simulink model "second_order_algorithm"  (R2020b)
settings: Solver=VariableStepAuto  StartTime=0.0  StopTime=4  RelTol=1e-3
undefined symbols (not defined in the file or in its folder): DiscIntNeverNeededParam
settings Model: Creator=martin  LastModifiedBy=martin

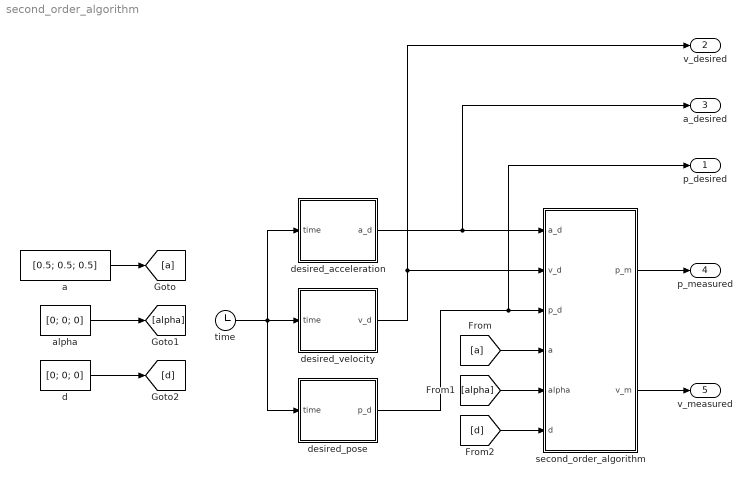
== system second_order_algorithm ==
  a : Constant  Value=[0.5; 0.5; 0.5]
  alpha : Constant  Value=[0; 0; 0]
  d : Constant  Value=[0; 0; 0]
  desired_acceleration : Subsystem
  desired_pose : Subsystem
  desired_velocity : Subsystem
  second_order_algorithm : Subsystem
  time : Clock
  p_desired : Outport
  v_desired : Outport  Port=2
  a_desired : Outport  Port=3
  p_measured : Outport  Port=4
  v_measured : Outport  Port=5
  wires:
  time/1 -> desired_pose/1(time), desired_velocity/1(time), desired_acceleration/1(time)
  a/1 -> [a]
  alpha/1 -> [alpha]
  d/1 -> [d]
  desired_velocity/1(v_d) -> second_order_algorithm/2(v_d), v_desired/1
  desired_pose/1(p_d) -> second_order_algorithm/3(p_d), p_desired/1
  [a] -> second_order_algorithm/4(a)
  [alpha] -> second_order_algorithm/5(alpha)
  [d] -> second_order_algorithm/6(d)
  second_order_algorithm/1(p_m) -> p_measured/1
  second_order_algorithm/2(v_m) -> v_measured/1
  desired_acceleration/1(a_d) -> second_order_algorithm/1(a_d), a_desired/1

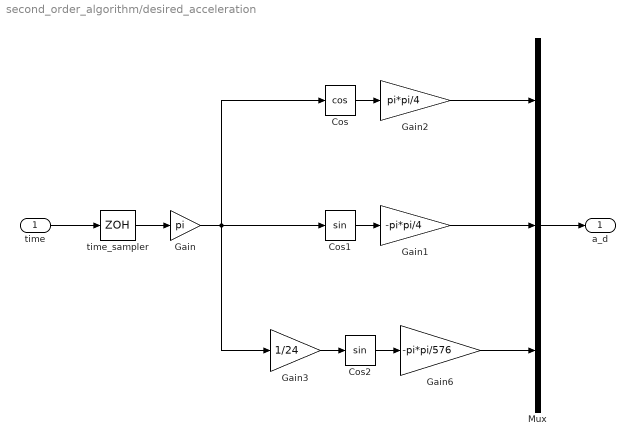
== system second_order_algorithm/desired_acceleration ==
  time : Inport
  Cos : Trigonometry  Operator=cos
  Cos1 : Trigonometry
  Cos2 : Trigonometry
  Gain : Gain  Gain=pi
  Gain1 : Gain  Gain=-pi*pi/4
  Gain2 : Gain  Gain=pi*pi/4
  Gain3 : Gain  Gain=1/24
  Gain6 : Gain  Gain=-pi*pi/576
  Mux : Mux  Inputs=3
  time_sampler : ZeroOrderHold  SampleTime=1e-3
  a_d : Outport
  wires:
  Mux/1 -> a_d/1
  Gain2/1 -> Mux/1
  Gain1/1 -> Mux/2
  time_sampler/1 -> Gain/1
  time/1 -> time_sampler/1
  Gain/1 -> Cos/1, Cos1/1, Gain3/1
  Cos/1 -> Gain2/1
  Cos1/1 -> Gain1/1
  Gain3/1 -> Cos2/1
  Cos2/1 -> Gain6/1
  Gain6/1 -> Mux/3

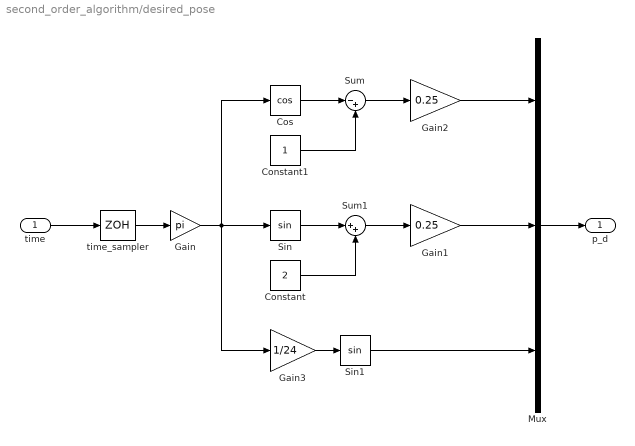
== system second_order_algorithm/desired_pose ==
  time : Inport
  Constant : Constant  Value=2
  Constant1 : Constant
  Cos : Trigonometry  Operator=cos
  Gain : Gain  Gain=pi
  Gain1 : Gain  Gain=0.25
  Gain2 : Gain  Gain=0.25
  Gain3 : Gain  Gain=1/24
  Mux : Mux  Inputs=3
  Sin : Trigonometry
  Sin1 : Trigonometry
  Sum : Sum  Inputs=|-+
  Sum1 : Sum  Inputs=|++
  time_sampler : ZeroOrderHold  SampleTime=1e-3
  p_d : Outport
  wires:
  Mux/1 -> p_d/1
  Cos/1 -> Sum/1
  Sum/1 -> Gain2/1
  Constant1/1 -> Sum/2
  Gain/1 -> Gain3/1, Sin/1, Cos/1
  Sin1/1 -> Mux/3
  Gain2/1 -> Mux/1
  Gain3/1 -> Sin1/1
  Gain1/1 -> Mux/2
  Sin/1 -> Sum1/1
  Constant/1 -> Sum1/2
  Sum1/1 -> Gain1/1
  time_sampler/1 -> Gain/1
  time/1 -> time_sampler/1

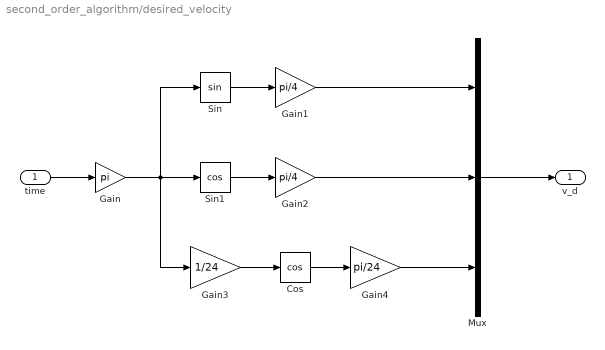
== system second_order_algorithm/desired_velocity ==
  time : Inport
  Cos : Trigonometry  Operator=cos
  Gain : Gain  Gain=pi
  Gain1 : Gain  Gain=pi/4
  Gain2 : Gain  Gain=pi/4
  Gain3 : Gain  Gain=1/24
  Gain4 : Gain  Gain=pi/24
  Mux : Mux  Inputs=3
  Sin : Trigonometry
  Sin1 : Trigonometry  Operator=cos
  v_d : Outport
  wires:
  time/1 -> Gain/1
  Gain/1 -> Gain3/1, Sin1/1, Sin/1
  Sin/1 -> Gain1/1
  Sin1/1 -> Gain2/1
  Gain3/1 -> Cos/1
  Cos/1 -> Gain4/1
  Gain1/1 -> Mux/1
  Gain2/1 -> Mux/2
  Mux/1 -> v_d/1
  Gain4/1 -> Mux/3

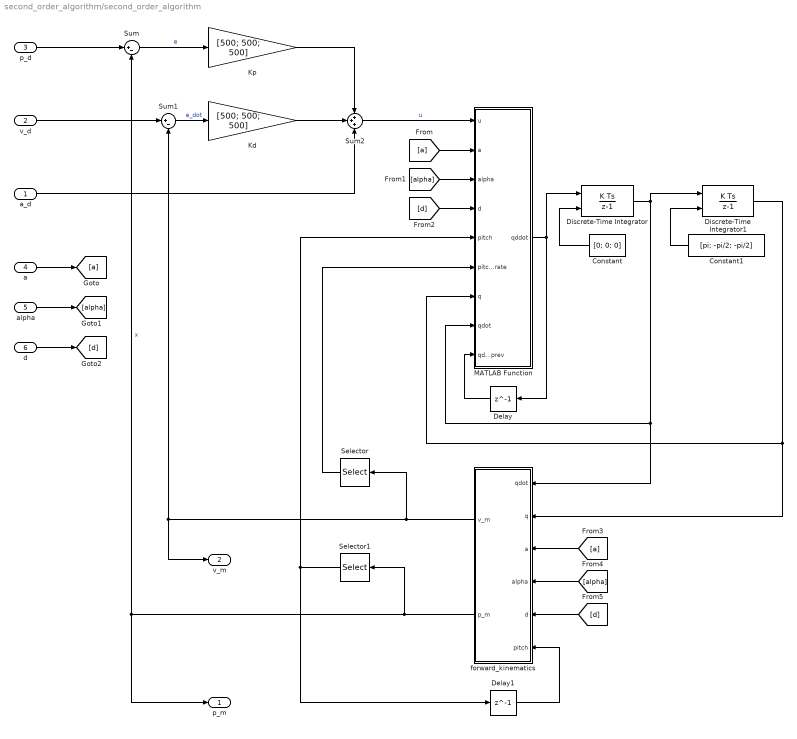
== system second_order_algorithm/second_order_algorithm ==
  a_d : Inport
  v_d : Inport  Port=2
  p_d : Inport  Port=3
  a : Inport  Port=4
  alpha : Inport  Port=5
  d : Inport  Port=6
  Constant : Constant  Value=[0; 0; 0]
  Constant1 : Constant  Value=[pi; -pi/2; -pi/2]
  Delay : Delay  DelayLength=1
  Delay1 : Delay  DelayLength=1
  Discrete-Time Integrator : DiscreteIntegrator  InitialConditionSource=external  SampleTime=1e-3  ICPrevOutput=DiscIntNeverNeededParam  ICPrevScaledInput=DiscIntNeverNeededParam
  Discrete-Time Integrator1 : DiscreteIntegrator  InitialConditionSource=external  SampleTime=1e-3  ICPrevOutput=DiscIntNeverNeededParam  ICPrevScaledInput=DiscIntNeverNeededParam
  Kd : Gain  Gain=[500; 500; 500]
  Kp : Gain  Gain=[500; 500; 500]
  MATLAB Function : MATLAB Function  TreatAsAtomicUnit=on
  Selector : Selector  InputPortWidth=3  IndexOptions=Index vector (dialog)  Indices=[3]  OutputSizes=1
  Selector1 : Selector  InputPortWidth=3  IndexOptions=Index vector (dialog)  Indices=[3]  OutputSizes=1
  Sum : Sum  Inputs=|+-
  Sum1 : Sum  Inputs=|+-
  Sum2 : Sum  Inputs=+++
  forward_kinematics : MATLAB Function  TreatAsAtomicUnit=on
  p_m : Outport
  v_m : Outport  Port=2
  wires:
  [d] -> forward_kinematics/5(d)
  [a] -> forward_kinematics/3(a)
  [alpha] -> forward_kinematics/4(alpha)
  Sum/1 -> Kp/1  "e"
  p_d/1 -> Sum/1
  v_d/1 -> Sum1/1
  Sum1/1 -> Kd/1  "e_dot"
  Kp/1 -> Sum2/1
  a_d/1 -> Sum2/3
  Kd/1 -> Sum2/2
  Sum2/1 -> MATLAB Function/1(u)  "u"
  MATLAB Function/1(qddot) -> Delay/1, Discrete-Time Integrator/1
  Constant/1 -> Discrete-Time Integrator/2
  Discrete-Time Integrator/1 -> forward_kinematics/1(qdot), MATLAB Function/8(qdot), Discrete-Time Integrator1/1
  Constant1/1 -> Discrete-Time Integrator1/2
  [alpha] -> MATLAB Function/3(alpha)
  [a] -> MATLAB Function/2(a)
  [d] -> MATLAB Function/4(d)
  Delay/1 -> MATLAB Function/9(qddot_prev)
  Discrete-Time Integrator1/1 -> forward_kinematics/2(q), MATLAB Function/7(q)
  forward_kinematics/1(v_m) -> Selector/1, v_m/1, Sum1/2
  forward_kinematics/2(p_m) -> Selector1/1, p_m/1, Sum/2  "x"
  Selector/1 -> MATLAB Function/6(pitch_rate)
  Selector1/1 -> Delay1/1, MATLAB Function/5(pitch)
  Delay1/1 -> forward_kinematics/6(pitch)
  alpha/1 -> [alpha]
  a/1 -> [a]
  d/1 -> [d]

== matlab function second_order_algorithm/forward_kinematics ==
  data: v_m output; qdot input; q input; a input; alpha input; d input; p_m output; pitch input
function [v_m, p_m] = fcn(qdot, q, a, alpha, d, pitch)
joint_type = ['r'; 'r'; 'r'];

s = forward_kinematics(joint_type, q, a, alpha, d);

J = s.analytical_jacobian(0, pitch);
J_min = [J(1:2,:); J(6,:)];
v_m = J_min*qdot;

x = s.end_effector_pose();
p_m = [x(1:2,:); x(6,:)];

== matlab function second_order_algorithm/MATLAB Function ==
  data: u input size=[3,1]; a input; alpha input; d input; pitch input; pitch_rate input; qddot output size=[3,1]; q input size=[3,1]; qdot input size=[3,1]; qddot_prev input size=[3,1]
function qddot = fcn(u, a, alpha, d, pitch, pitch_rate, q, qdot, qddot_prev)

joint_type = ['r'; 'r'; 'r'];

s = forward_kinematics(joint_type, q, a, alpha, d);

J = s.analytical_jacobian(0, pitch);

J_min = [J(1:2,:); J(6,:)];

J_inv = (transpose(J_min)/(J_min*transpose(J_min)));

[a1, a2, a3] = split_into_three(a);
[q1, q2, q3] = split_into_three(q);
[qdot1, qdot2, qdot3] = split_into_three(qdot);

Jdot = Jdot_RRR(a1,a2,a3,q1,q2,q3,qdot1,qdot2,qdot3,pitch,pitch_rate);
Jdot_min = [Jdot(1:2,:); Jdot(6,:)];

qddot = J_inv*(u - Jdot_min*qdot) + (eye(3,3) - J_inv*J_min)*qddot_prev;

    function [x1, x2, x3] = split_into_three(x)
        x1 = x(1,1);
        x2 = x(2,1);
        x3 = x(3,1);
    end
end
